simulink model "cruisecontrol"  (Simulink 5.0)
settings: Solver=ode45  StartTime=0.0  StopTime=10.0  RelTol=1e-3
settings Model: ExecutionOrder=on  LastModifiedBy=eal  BooleanDataType=off  OptimizeBlockIOStorage=off

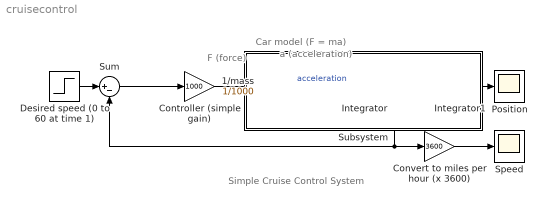
== system cruisecontrol ==
  note: Simple Cruise Control System
  note: Car model (F = ma)
  note: a
      | (acceleration)
  note: F
      | (force)
  "  Controller (simple gain)" : Gain  Gain=1000  SaturateOnIntegerOverflow=on
  " Convert to miles per hour (x 3600)" : Gain  Gain=3600  SaturateOnIntegerOverflow=on
  1/mass : Gain  Gain=1/1000  SaturateOnIntegerOverflow=on
  Desired speed (0 to 60 at time 1) : Step  After=60/3600  SampleTime=0
  Integrator : Integrator
  Integrator1 : Integrator
  Position : Scope
      settings: TimeRange=10  YMin=0  YMax=0.2
  Speed : Scope
      settings: TimeRange=10  YMin=0  YMax=0.02
  Subsystem : Subsystem
  Sum : Sum  Inputs=|+-  SaturateOnIntegerOverflow=on  InputSameDT=on
  wires:
  Desired speed (0 to 60 at time 1)/1 -> Sum/1
  Integrator1/1 -> Position/1
  Sum/1 -> "  Controller (simple gain)"/1
  Integrator/1 -> Integrator1/1, Sum/2, " Convert to miles per hour (x 3600)"/1
  "  Controller (simple gain)"/1 -> 1/mass/1
  1/mass/1 -> Integrator/1  "acceleration"
  " Convert to miles per hour (x 3600)"/1 -> Speed/1

== system cruisecontrol/Subsystem ==
